simulink model "imuentiljorgen"  (R2024a)
settings: Solver=ode45  StartTime=0.0  StopTime=inf  MaxStep=1e-2  MinStep=1e-4  RelTol=1e-3
InitFcn:
  | id_setup()
StartFcn:
  | c_id = evalin('base', "car_id");
  | g_id = evalin('base', "group_id");
  | mqttBasic(c_id,g_id);
StopFcn:
  | task = 1.1;
  | score = evalin('base', "score");
  | send_score(task,score);
libraries: init x2, read x1, send x1
settings Model: PacingRate=3  Creator=adriaeik  LastModifiedBy=adriaeik

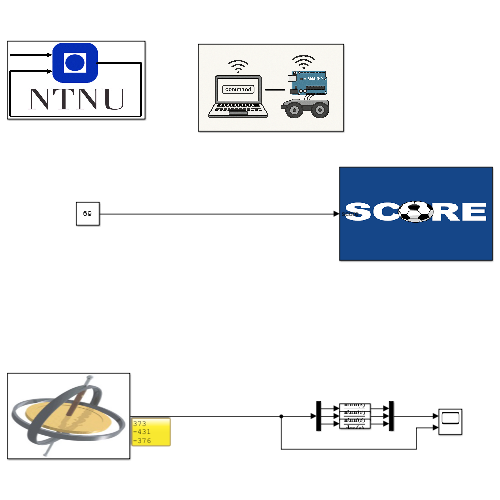
[thumbnail: Simulink's stored preview of the top-level diagram]
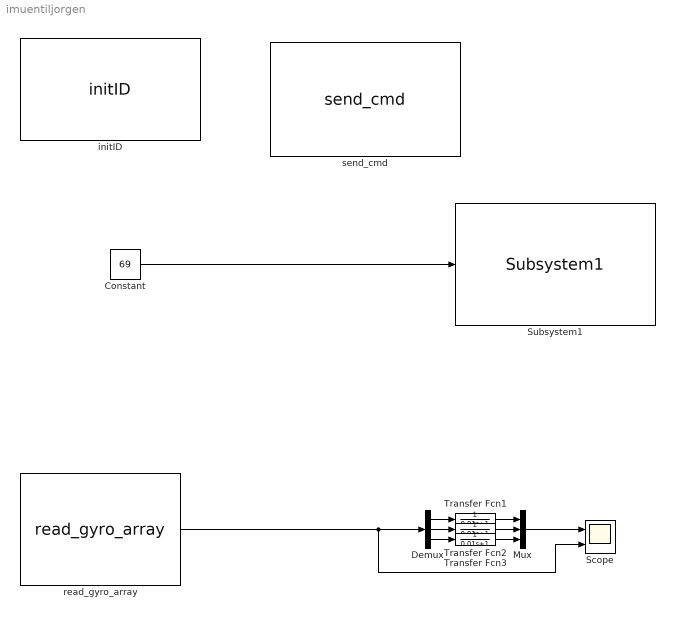
== system imuentiljorgen ==
  Constant : Constant  Value=69
  Demux : Demux  Outputs=3
  Mux : Mux  Inputs=3
  Scope : Scope  NumInputPorts=2
  Subsystem1 : init/Subsystem1  SystemSampleTime=-1  VariantActivationTime=update diagram  AllowFlexibleInterface=on  Latency=0  AutoFrameSizeCalculation=off
  Transfer Fcn1 : TransferFcn  Denominator=[0.01 1]
  Transfer Fcn2 : TransferFcn  Denominator=[0.01 1]
  Transfer Fcn3 : TransferFcn  Denominator=[0.01 1]
  initID : init/initID  carID=14  groupID=69
  read_gyro_array : read/read_gyro_array
  send_cmd : send/send_cmd  cmd=Stop
  wires:
  Constant/1 -> Subsystem1/1
  read_gyro_array/1 -> Scope/2, Demux/1
  Demux/1 -> Transfer Fcn1/1
  Transfer Fcn1/1 -> Mux/1
  Demux/2 -> Transfer Fcn2/1
  Transfer Fcn2/1 -> Mux/2
  Demux/3 -> Transfer Fcn3/1
  Transfer Fcn3/1 -> Mux/3
  Mux/1 -> Scope/1
